simulink model "TST_HPUn_QntBalInjLim"  (R2016b)
settings: Solver=FixedStepDiscrete  StartTime=0.0  StopTime=simTime  FixedStep=sampleTime  RelTol=1e-3
values from neighbouring files (symbols this model uses):
  testCase = 1    [initTST_HPUn_QntBalInjLim_001.m]    (also in initTST_HPUn_QntBalInjLim_002.m = 2)
libraries: simulink x7, UnitTest_Lib x4
settings Model: Creator=zhengjinyan  LastModifiedBy=zhengjinyan
settings DebuggingCC: SignalRangeChecking=error

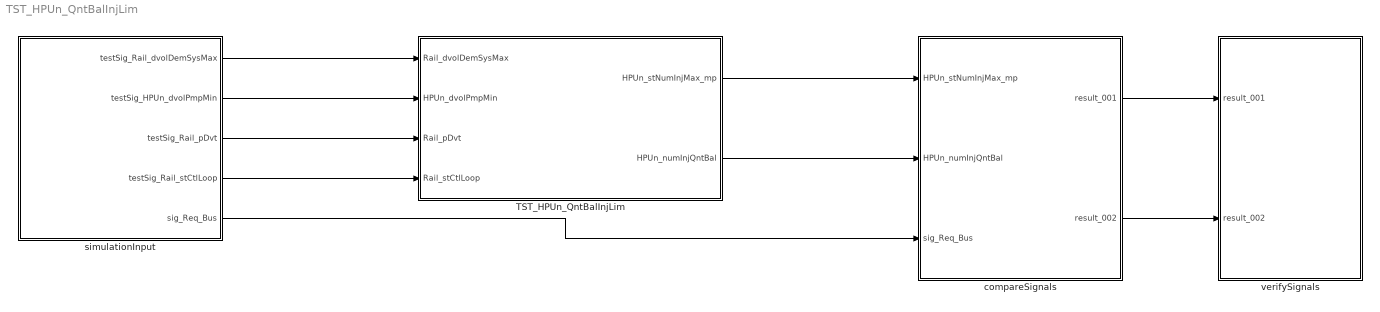
== system TST_HPUn_QntBalInjLim ==
  TST_HPUn_QntBalInjLim : Subsystem
  compareSignals : Subsystem
  simulationInput : Subsystem
  verifySignals : Subsystem
  wires:
  simulationInput/1(testSig_Rail_dvolDemSysMax) -> TST_HPUn_QntBalInjLim/1(Rail_dvolDemSysMax)
  simulationInput/2(testSig_HPUn_dvolPmpMin) -> TST_HPUn_QntBalInjLim/2(HPUn_dvolPmpMin)
  simulationInput/3(testSig_Rail_pDvt) -> TST_HPUn_QntBalInjLim/3(Rail_pDvt)
  simulationInput/4(testSig_Rail_stCtlLoop) -> TST_HPUn_QntBalInjLim/4(Rail_stCtlLoop)
  TST_HPUn_QntBalInjLim/1(HPUn_stNumInjMax_mp) -> compareSignals/1(HPUn_stNumInjMax_mp)
  TST_HPUn_QntBalInjLim/2(HPUn_numInjQntBal) -> compareSignals/2(HPUn_numInjQntBal)
  simulationInput/5(sig_Req_Bus) -> compareSignals/3(sig_Req_Bus)
  compareSignals/1(result_001) -> verifySignals/1(result_001)
  compareSignals/2(result_002) -> verifySignals/2(result_002)

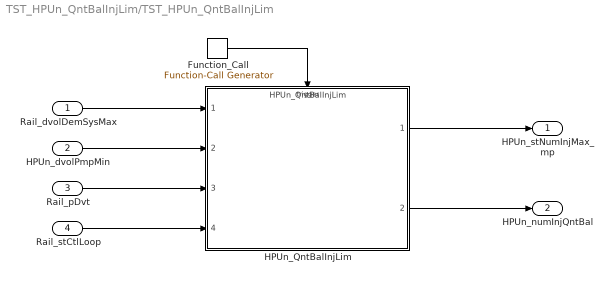
== system TST_HPUn_QntBalInjLim/TST_HPUn_QntBalInjLim ==
  Rail_dvolDemSysMax : Inport
  HPUn_dvolPmpMin : Inport  Port=2
  Rail_pDvt : Inport  Port=3
  Rail_stCtlLoop : Inport  Port=4
  Function_Call : simulink/Ports & Subsystems/Function-Call Generator  sample_time=sampleTime  numberOfIterations=1
  HPUn_QntBalInjLim : ModelReference  ModelNameDialog=HPUn_QntBalInjLim  SimulationMode=Normal  ModelReferenceVersion=1.18  TriggerPortName=function  TriggerPortTriggerType=function-call  TriggerPortStatesWhenEnabling=held
  HPUn_stNumInjMax_mp : Outport
  HPUn_numInjQntBal : Outport  Port=2
  wires:
  Function_Call/1 -> HPUn_QntBalInjLim/Trigger
  Rail_dvolDemSysMax/1 -> HPUn_QntBalInjLim/1
  HPUn_dvolPmpMin/1 -> HPUn_QntBalInjLim/2
  Rail_pDvt/1 -> HPUn_QntBalInjLim/3
  Rail_stCtlLoop/1 -> HPUn_QntBalInjLim/4
  HPUn_QntBalInjLim/1 -> HPUn_stNumInjMax_mp/1
  HPUn_QntBalInjLim/2 -> HPUn_numInjQntBal/1

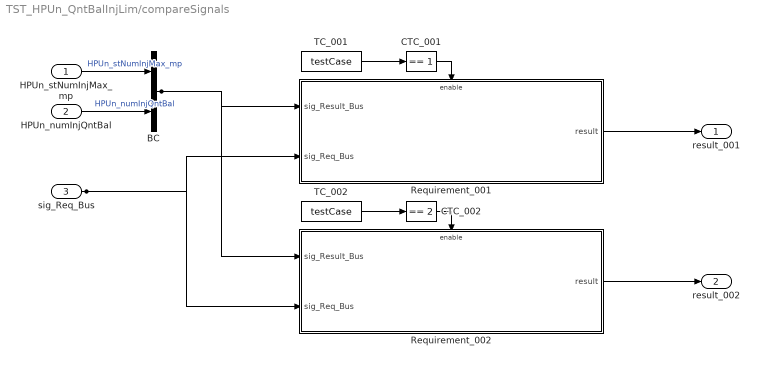
== system TST_HPUn_QntBalInjLim/compareSignals ==
  HPUn_stNumInjMax_mp : Inport
  HPUn_numInjQntBal : Inport  Port=2
  sig_Req_Bus : Inport  Port=3
  BC : BusCreator  Inputs=2
  CTC_001 : simulink/Logic and Bit Operations/Compare To Constant  relop===  const=1  OutDataTypeStr=boolean
  CTC_002 : simulink/Logic and Bit Operations/Compare To Constant  relop===  const=2  OutDataTypeStr=boolean
  Requirement_001 : Subsystem
  Requirement_002 : Subsystem
  TC_001 : Constant  Value=testCase
  TC_002 : Constant  Value=testCase
  result_001 : Outport
  result_002 : Outport  Port=2
  wires:
  HPUn_stNumInjMax_mp/1 -> BC/1  "HPUn_stNumInjMax_mp"
  HPUn_numInjQntBal/1 -> BC/2  "HPUn_numInjQntBal"
  TC_001/1 -> CTC_001/1
  CTC_001/1 -> Requirement_001/Enable
  sig_Req_Bus/1 -> Requirement_001/2(sig_Req_Bus), Requirement_002/2(sig_Req_Bus)
  BC/1 -> Requirement_001/1(sig_Result_Bus), Requirement_002/1(sig_Result_Bus)
  Requirement_001/1(result) -> result_001/1
  TC_002/1 -> CTC_002/1
  CTC_002/1 -> Requirement_002/Enable
  Requirement_002/1(result) -> result_002/1

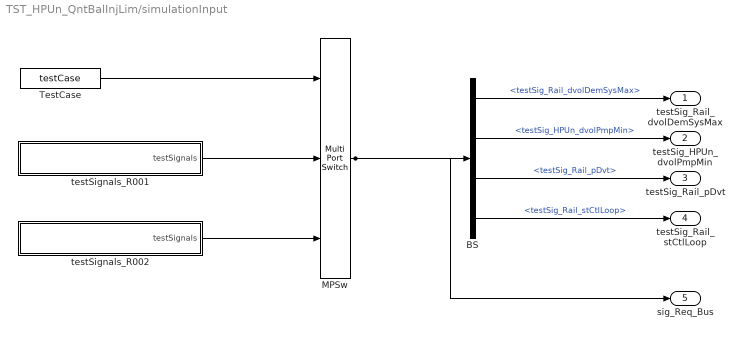
== system TST_HPUn_QntBalInjLim/simulationInput ==
  BS : BusSelector  OutputSignals=testSig_Rail_dvolDemSysMax,testSig_HPUn_dvolPmpMin,testSig_Rail_pDvt,testSig_Rail_stCtlLoop
  MPSw : MultiPortSwitch  Inputs=2  SaturateOnIntegerOverflow=on  InputSameDT=on
  TestCase : Constant  Value=testCase
  testSignals_R001 : Subsystem
  testSignals_R002 : Subsystem
  testSig_Rail_dvolDemSysMax : Outport
  testSig_HPUn_dvolPmpMin : Outport  Port=2
  testSig_Rail_pDvt : Outport  Port=3
  testSig_Rail_stCtlLoop : Outport  Port=4
  sig_Req_Bus : Outport  Port=5
  wires:
  BS/1 -> testSig_Rail_dvolDemSysMax/1  "<testSig_Rail_dvolDemSysMax>"
  BS/2 -> testSig_HPUn_dvolPmpMin/1  "<testSig_HPUn_dvolPmpMin>"
  BS/3 -> testSig_Rail_pDvt/1  "<testSig_Rail_pDvt>"
  BS/4 -> testSig_Rail_stCtlLoop/1  "<testSig_Rail_stCtlLoop>"
  MPSw/1 -> BS/1, sig_Req_Bus/1
  TestCase/1 -> MPSw/1
  testSignals_R001/1(testSignals) -> MPSw/2
  testSignals_R002/1(testSignals) -> MPSw/3

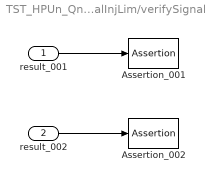
== system TST_HPUn_QntBalInjLim/verifySignals ==
  result_001 : Inport
  result_002 : Inport  Port=2
  Assertion_001 : Assertion  Enabled=off
  Assertion_002 : Assertion  Enabled=off
  wires:
  result_001/1 -> Assertion_001/1
  result_002/1 -> Assertion_002/1

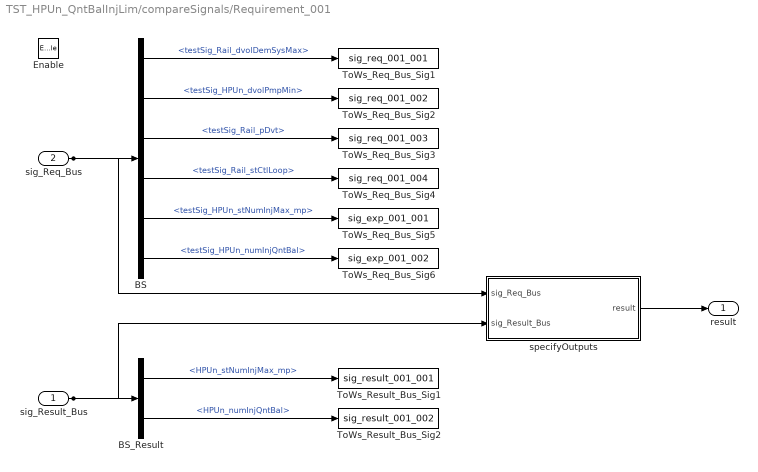
== system TST_HPUn_QntBalInjLim/compareSignals/Requirement_001 ==
  sig_Result_Bus : Inport
  sig_Req_Bus : Inport  Port=2
  Enable : EnablePort
  BS : BusSelector  OutputSignals=testSig_Rail_dvolDemSysMax,testSig_HPUn_dvolPmpMin,testSig_Rail_pDvt,testSig_Rail_stCtlLoop,testSig_HPUn_stNumInjMax_mp,testSig_HPUn_numInjQntBal
  BS_Result : BusSelector  OutputSignals=HPUn_stNumInjMax_mp,HPUn_numInjQntBal
  ToWs_Req_Bus_Sig1 : ToWorkspace  VariableName=sig_req_001_001  SaveFormat=Structure With Time
  ToWs_Req_Bus_Sig2 : ToWorkspace  VariableName=sig_req_001_002  SaveFormat=Structure With Time
  ToWs_Req_Bus_Sig3 : ToWorkspace  VariableName=sig_req_001_003  SaveFormat=Structure With Time
  ToWs_Req_Bus_Sig4 : ToWorkspace  VariableName=sig_req_001_004  SaveFormat=Structure With Time
  ToWs_Req_Bus_Sig5 : ToWorkspace  VariableName=sig_exp_001_001  SaveFormat=Structure With Time
  ToWs_Req_Bus_Sig6 : ToWorkspace  VariableName=sig_exp_001_002  SaveFormat=Structure With Time
  ToWs_Result_Bus_Sig1 : ToWorkspace  VariableName=sig_result_001_001  SaveFormat=Structure With Time
  ToWs_Result_Bus_Sig2 : ToWorkspace  VariableName=sig_result_001_002  SaveFormat=Structure With Time
  specifyOutputs : Subsystem
  result : Outport
  wires:
  sig_Req_Bus/1 -> BS/1, specifyOutputs/1(sig_Req_Bus)
  BS/1 -> ToWs_Req_Bus_Sig1/1  "<testSig_Rail_dvolDemSysMax>"
  BS/2 -> ToWs_Req_Bus_Sig2/1  "<testSig_HPUn_dvolPmpMin>"
  BS/3 -> ToWs_Req_Bus_Sig3/1  "<testSig_Rail_pDvt>"
  BS/4 -> ToWs_Req_Bus_Sig4/1  "<testSig_Rail_stCtlLoop>"
  BS/5 -> ToWs_Req_Bus_Sig5/1  "<testSig_HPUn_stNumInjMax_mp>"
  BS/6 -> ToWs_Req_Bus_Sig6/1  "<testSig_HPUn_numInjQntBal>"
  sig_Result_Bus/1 -> BS_Result/1, specifyOutputs/2(sig_Result_Bus)
  BS_Result/1 -> ToWs_Result_Bus_Sig1/1  "<HPUn_stNumInjMax_mp>"
  BS_Result/2 -> ToWs_Result_Bus_Sig2/1  "<HPUn_numInjQntBal>"
  specifyOutputs/1(result) -> result/1

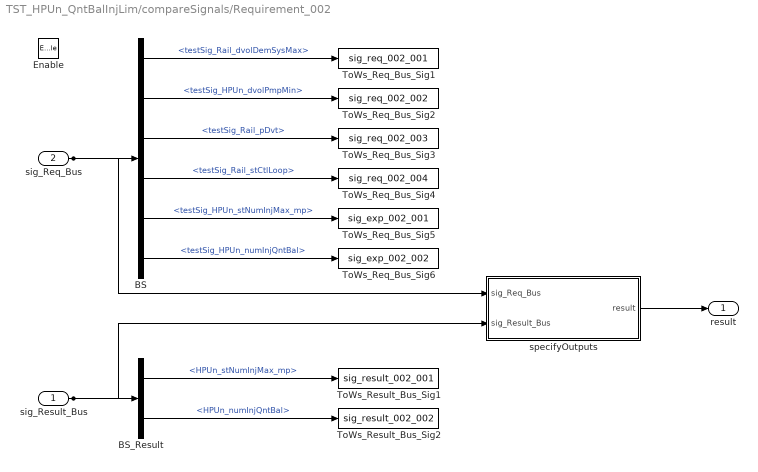
== system TST_HPUn_QntBalInjLim/compareSignals/Requirement_002 ==
  sig_Result_Bus : Inport
  sig_Req_Bus : Inport  Port=2
  Enable : EnablePort
  BS : BusSelector  OutputSignals=testSig_Rail_dvolDemSysMax,testSig_HPUn_dvolPmpMin,testSig_Rail_pDvt,testSig_Rail_stCtlLoop,testSig_HPUn_stNumInjMax_mp,testSig_HPUn_numInjQntBal
  BS_Result : BusSelector  OutputSignals=HPUn_stNumInjMax_mp,HPUn_numInjQntBal
  ToWs_Req_Bus_Sig1 : ToWorkspace  VariableName=sig_req_002_001  SaveFormat=Structure With Time
  ToWs_Req_Bus_Sig2 : ToWorkspace  VariableName=sig_req_002_002  SaveFormat=Structure With Time
  ToWs_Req_Bus_Sig3 : ToWorkspace  VariableName=sig_req_002_003  SaveFormat=Structure With Time
  ToWs_Req_Bus_Sig4 : ToWorkspace  VariableName=sig_req_002_004  SaveFormat=Structure With Time
  ToWs_Req_Bus_Sig5 : ToWorkspace  VariableName=sig_exp_002_001  SaveFormat=Structure With Time
  ToWs_Req_Bus_Sig6 : ToWorkspace  VariableName=sig_exp_002_002  SaveFormat=Structure With Time
  ToWs_Result_Bus_Sig1 : ToWorkspace  VariableName=sig_result_002_001  SaveFormat=Structure With Time
  ToWs_Result_Bus_Sig2 : ToWorkspace  VariableName=sig_result_002_002  SaveFormat=Structure With Time
  specifyOutputs : Subsystem
  result : Outport
  wires:
  sig_Req_Bus/1 -> BS/1, specifyOutputs/1(sig_Req_Bus)
  BS/1 -> ToWs_Req_Bus_Sig1/1  "<testSig_Rail_dvolDemSysMax>"
  BS/2 -> ToWs_Req_Bus_Sig2/1  "<testSig_HPUn_dvolPmpMin>"
  BS/3 -> ToWs_Req_Bus_Sig3/1  "<testSig_Rail_pDvt>"
  BS/4 -> ToWs_Req_Bus_Sig4/1  "<testSig_Rail_stCtlLoop>"
  BS/5 -> ToWs_Req_Bus_Sig5/1  "<testSig_HPUn_stNumInjMax_mp>"
  BS/6 -> ToWs_Req_Bus_Sig6/1  "<testSig_HPUn_numInjQntBal>"
  sig_Result_Bus/1 -> BS_Result/1, specifyOutputs/2(sig_Result_Bus)
  BS_Result/1 -> ToWs_Result_Bus_Sig1/1  "<HPUn_stNumInjMax_mp>"
  BS_Result/2 -> ToWs_Result_Bus_Sig2/1  "<HPUn_numInjQntBal>"
  specifyOutputs/1(result) -> result/1

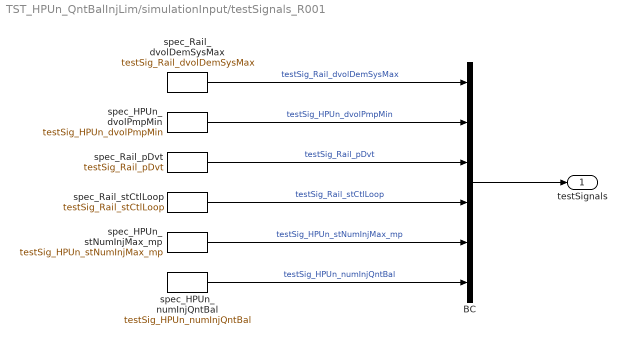
== system TST_HPUn_QntBalInjLim/simulationInput/testSignals_R001 ==
  BC : BusCreator  Inputs=6
  spec_HPUn_dvolPmpMin : FromWorkspace  VariableName=testSig_HPUn_dvolPmpMin  Interpolate=off  OutputAfterFinalValue=Holding final value
  spec_HPUn_numInjQntBal : FromWorkspace  VariableName=testSig_HPUn_numInjQntBal  Interpolate=off  OutputAfterFinalValue=Holding final value
  spec_HPUn_stNumInjMax_mp : FromWorkspace  VariableName=testSig_HPUn_stNumInjMax_mp  Interpolate=off  OutputAfterFinalValue=Holding final value
  spec_Rail_dvolDemSysMax : FromWorkspace  VariableName=testSig_Rail_dvolDemSysMax  Interpolate=off  OutputAfterFinalValue=Holding final value
  spec_Rail_pDvt : FromWorkspace  VariableName=testSig_Rail_pDvt  Interpolate=off  OutputAfterFinalValue=Holding final value
  spec_Rail_stCtlLoop : FromWorkspace  VariableName=testSig_Rail_stCtlLoop  Interpolate=off  OutputAfterFinalValue=Holding final value
  testSignals : Outport
  wires:
  BC/1 -> testSignals/1
  spec_Rail_dvolDemSysMax/1 -> BC/1  "testSig_Rail_dvolDemSysMax"
  spec_HPUn_dvolPmpMin/1 -> BC/2  "testSig_HPUn_dvolPmpMin"
  spec_Rail_pDvt/1 -> BC/3  "testSig_Rail_pDvt"
  spec_Rail_stCtlLoop/1 -> BC/4  "testSig_Rail_stCtlLoop"
  spec_HPUn_stNumInjMax_mp/1 -> BC/5  "testSig_HPUn_stNumInjMax_mp"
  spec_HPUn_numInjQntBal/1 -> BC/6  "testSig_HPUn_numInjQntBal"

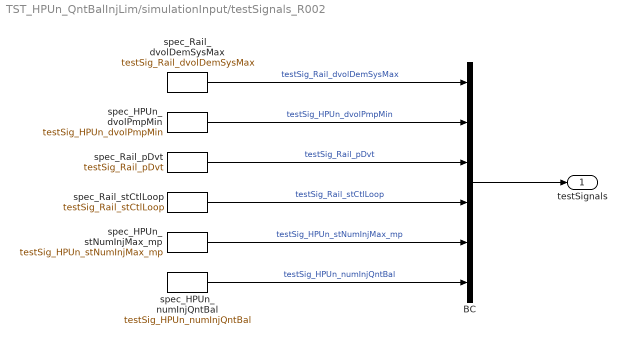
== system TST_HPUn_QntBalInjLim/simulationInput/testSignals_R002 ==
  BC : BusCreator  Inputs=6
  spec_HPUn_dvolPmpMin : FromWorkspace  VariableName=testSig_HPUn_dvolPmpMin  Interpolate=off  OutputAfterFinalValue=Holding final value
  spec_HPUn_numInjQntBal : FromWorkspace  VariableName=testSig_HPUn_numInjQntBal  Interpolate=off  OutputAfterFinalValue=Holding final value
  spec_HPUn_stNumInjMax_mp : FromWorkspace  VariableName=testSig_HPUn_stNumInjMax_mp  Interpolate=off  OutputAfterFinalValue=Holding final value
  spec_Rail_dvolDemSysMax : FromWorkspace  VariableName=testSig_Rail_dvolDemSysMax  Interpolate=off  OutputAfterFinalValue=Holding final value
  spec_Rail_pDvt : FromWorkspace  VariableName=testSig_Rail_pDvt  Interpolate=off  OutputAfterFinalValue=Holding final value
  spec_Rail_stCtlLoop : FromWorkspace  VariableName=testSig_Rail_stCtlLoop  Interpolate=off  OutputAfterFinalValue=Holding final value
  testSignals : Outport
  wires:
  BC/1 -> testSignals/1
  spec_Rail_dvolDemSysMax/1 -> BC/1  "testSig_Rail_dvolDemSysMax"
  spec_HPUn_dvolPmpMin/1 -> BC/2  "testSig_HPUn_dvolPmpMin"
  spec_Rail_pDvt/1 -> BC/3  "testSig_Rail_pDvt"
  spec_Rail_stCtlLoop/1 -> BC/4  "testSig_Rail_stCtlLoop"
  spec_HPUn_stNumInjMax_mp/1 -> BC/5  "testSig_HPUn_stNumInjMax_mp"
  spec_HPUn_numInjQntBal/1 -> BC/6  "testSig_HPUn_numInjQntBal"

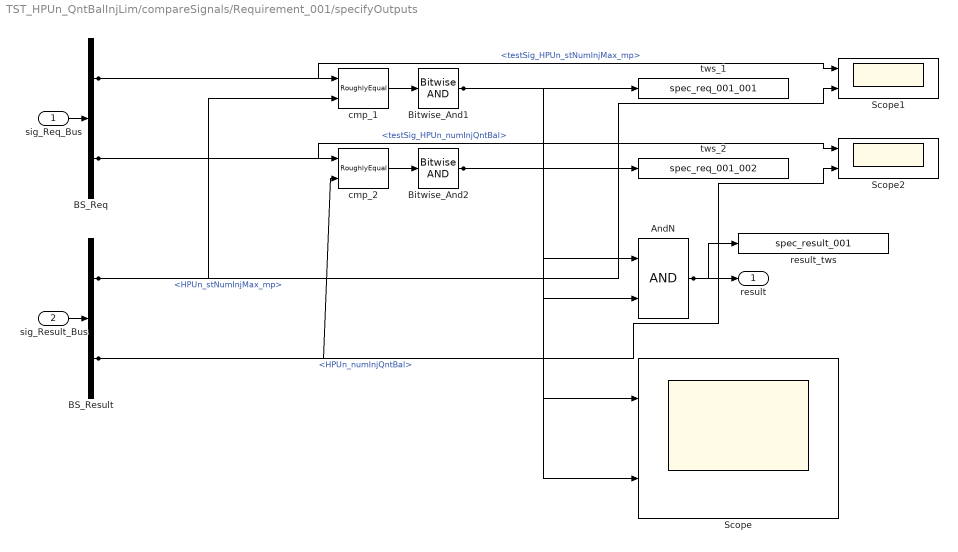
== system TST_HPUn_QntBalInjLim/compareSignals/Requirement_001/specifyOutputs ==
  sig_Req_Bus : Inport
  sig_Result_Bus : Inport  Port=2
  AndN : Logic
  BS_Req : BusSelector  OutputSignals=testSig_HPUn_stNumInjMax_mp,testSig_HPUn_numInjQntBal
  BS_Result : BusSelector  OutputSignals=HPUn_stNumInjMax_mp,HPUn_numInjQntBal
  Bitwise_And1 : simulink/Logic and Bit Operations/Bitwise Operator  logicop=AND  UseBitMask=off  BitMask=bin2dec('11011001')  BitMaskRealWorld=Stored Integer
  Bitwise_And2 : simulink/Logic and Bit Operations/Bitwise Operator  logicop=AND  UseBitMask=off  BitMask=bin2dec('11011001')  BitMaskRealWorld=Stored Integer
  Scope : Scope  NumInputPorts=2
  Scope1 : Scope  NumInputPorts=2
  Scope2 : Scope  NumInputPorts=2
  cmp_1 : UnitTest_Lib/RoughlyEqual  slope=0.1
  cmp_2 : UnitTest_Lib/RoughlyEqual  slope=0.1
  result_tws : ToWorkspace  VariableName=spec_result_001
  tws_1 : ToWorkspace  VariableName=spec_req_001_001
  tws_2 : ToWorkspace  VariableName=spec_req_001_002
  result : Outport
  wires:
  sig_Req_Bus/1 -> BS_Req/1
  sig_Result_Bus/1 -> BS_Result/1
  AndN/1 -> result/1, result_tws/1
  BS_Req/1 -> cmp_1/1, Scope1/1  "<testSig_HPUn_stNumInjMax_mp>"
  BS_Result/1 -> cmp_1/2, Scope1/2  "<HPUn_stNumInjMax_mp>"
  cmp_1/1 -> Bitwise_And1/1
  Bitwise_And1/1 -> tws_1/1, AndN/1, Scope/1
  BS_Req/2 -> cmp_2/1, Scope2/1  "<testSig_HPUn_numInjQntBal>"
  BS_Result/2 -> cmp_2/2, Scope2/2  "<HPUn_numInjQntBal>"
  cmp_2/1 -> Bitwise_And2/1
  Bitwise_And2/1 -> tws_2/1, AndN/2, Scope/2

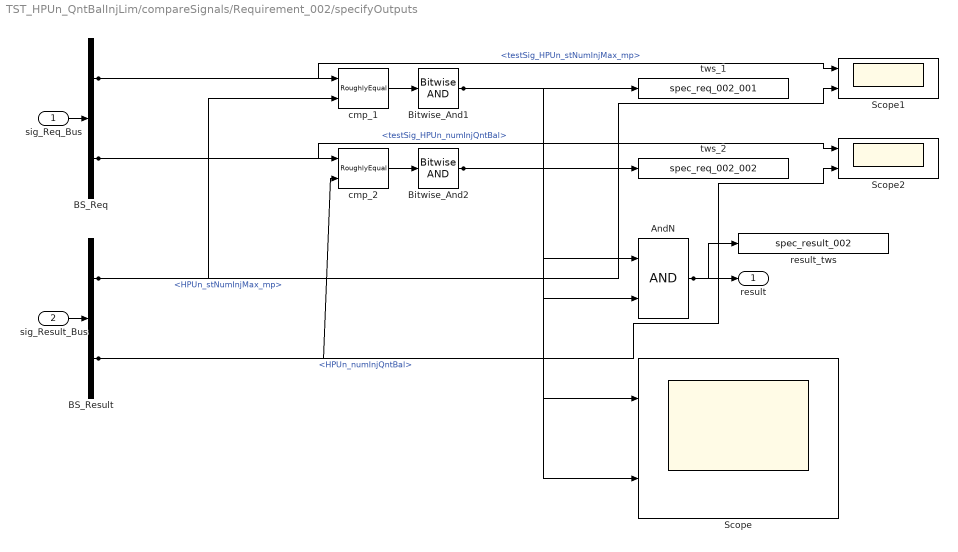
== system TST_HPUn_QntBalInjLim/compareSignals/Requirement_002/specifyOutputs ==
  sig_Req_Bus : Inport
  sig_Result_Bus : Inport  Port=2
  AndN : Logic
  BS_Req : BusSelector  OutputSignals=testSig_HPUn_stNumInjMax_mp,testSig_HPUn_numInjQntBal
  BS_Result : BusSelector  OutputSignals=HPUn_stNumInjMax_mp,HPUn_numInjQntBal
  Bitwise_And1 : simulink/Logic and Bit Operations/Bitwise Operator  logicop=AND  UseBitMask=off  BitMask=bin2dec('11011001')  BitMaskRealWorld=Stored Integer
  Bitwise_And2 : simulink/Logic and Bit Operations/Bitwise Operator  logicop=AND  UseBitMask=off  BitMask=bin2dec('11011001')  BitMaskRealWorld=Stored Integer
  Scope : Scope  NumInputPorts=2
  Scope1 : Scope  NumInputPorts=2
  Scope2 : Scope  NumInputPorts=2
  cmp_1 : UnitTest_Lib/RoughlyEqual  slope=0.1
  cmp_2 : UnitTest_Lib/RoughlyEqual  slope=0.1
  result_tws : ToWorkspace  VariableName=spec_result_002
  tws_1 : ToWorkspace  VariableName=spec_req_002_001
  tws_2 : ToWorkspace  VariableName=spec_req_002_002
  result : Outport
  wires:
  sig_Req_Bus/1 -> BS_Req/1
  sig_Result_Bus/1 -> BS_Result/1
  AndN/1 -> result/1, result_tws/1
  BS_Req/1 -> cmp_1/1, Scope1/1  "<testSig_HPUn_stNumInjMax_mp>"
  BS_Result/1 -> cmp_1/2, Scope1/2  "<HPUn_stNumInjMax_mp>"
  cmp_1/1 -> Bitwise_And1/1
  Bitwise_And1/1 -> tws_1/1, AndN/1, Scope/1
  BS_Req/2 -> cmp_2/1, Scope2/1  "<testSig_HPUn_numInjQntBal>"
  BS_Result/2 -> cmp_2/2, Scope2/2  "<HPUn_numInjQntBal>"
  cmp_2/1 -> Bitwise_And2/1
  Bitwise_And2/1 -> tws_2/1, AndN/2, Scope/2
